simulink model "SPGF_FSK_0000_R2022b"  (R2022b)
settings: Solver=ode4  StartTime=0.0  StopTime=1.4  FixedStep=50e-6/50  RelTol=1e-3  EnableMultiTasking=on
undefined symbols (not defined in the file): D11, Delta
libraries: spsSeriesRLCBranchLib x1646, spsGroundLib x360, spsStairGeneratorLib x147, spsIdealSwitchLib x145, spsCurrentMeasurementLib x145, spsUniversalBridgeLib x76, spsThreePhaseSeriesRLCLoadLib x57, simulink x45, spsBistableLib x36, spsSequenceAnalyzerLib x31, spsThreePhaseParallelRLCLoadLib x20, spsThreePhaseTransformerTwoWindingsLib x20
(part 25 of 40)

== system SPGF_FSK_0000_R2022b/W33/DPL ==
  Ccs2/1 : spsSeriesRLCBranchLib/Series RLC Branch  LConnTagsString=__new0  RConnTagsString=__new0  BranchType=R  Resistance=-Rg_matrix(3,4)*2  Inductance=1e-3  SetiL0=off  InitialCurrent=0  Capacitance=Rg_matrix(3,4)*2  Setx0=off  InitialVoltage=0  Measurements=None
  Ccs2/3 : spsSeriesRLCBranchLib/Series RLC Branch  LConnTagsString=__new0  RConnTagsString=__new0  BranchType=R  Resistance=-Rg_matrix(3,4)*2  Inductance=1e-3  SetiL0=off  InitialCurrent=0  Capacitance=Rg_matrix(3,4)*2  Setx0=off  InitialVoltage=0  Measurements=None
  Ccs3/1 : spsSeriesRLCBranchLib/Series RLC Branch  LConnTagsString=__new0  RConnTagsString=__new0  BranchType=R  Resistance=-Rg_matrix(5,6)*2  Inductance=1e-3  SetiL0=off  InitialCurrent=0  Capacitance=-C_matrix(5,6)/2  Setx0=off  InitialVoltage=0  Measurements=None
  Ccs3/3 : spsSeriesRLCBranchLib/Series RLC Branch  LConnTagsString=__new0  RConnTagsString=__new0  BranchType=R  Resistance=-Rg_matrix(5,6)*2  Inductance=1e-3  SetiL0=off  InitialCurrent=0  Capacitance=-C_matrix(5,6)/2  Setx0=off  InitialVoltage=0  Measurements=None
  DPL : spsDistributedParametersLineLib/Distributed Parameters Line  Phases=6  Length=LineLength  Frequency=Frequency  Resistance=R_matrix  Inductance=L_matrix  Capacitance=C_matrix  x1=[-2.15e-05 -1.53051007031569 0 -12.0034457369496 0 0 -8990.94401290029;-2.1e-05 -1.53094778670127 0 -12.0068977094404 0 0 -8990.15397169475;-2.05e-05 -1.53138546531224 0 -12.010349385673 0 0 -8989.36370866606;-2e-05 -1.53182310613778 0 -12.013800765562 0 0 -8988.5732238337;-1.95e-05 -1.5322607091671 0 -12.0172518490225 0 0 -8987.78251721719;-1.9e-05 -1.5326982743894 0 -12.0207026359691 0 0 -8986.99158883604;-1.85e-05 -1.53313580179389 0 -12.0241531263167 0 0 -8986.20043870976;-1.8e-05 -1.53357329136977 0 -12.0276033199803 0 0 -8985.40906685787;-1.75e-05 -1.53401074310624 0 -12.0310532168746 0 0 -8984.6174732999;-1.7e-05 -1.53444815699252 0 -12.0345028169147 0 0 -8983.82565805538;-1.65e-05 -1.53488553301781 0 -12.0379521200152 0 0 -8983.03362114385;-1.6e-05 -1.53532287117131 0 -12.0414011260912 0 0 -8982.24136258485;-1.55e-05 -1.53576017144224 0 -12.0448498350576 0 0 -8981.44888239792;-1.5e-05 -1.53619743381981 0 -12.0482982468291 0 0 -8980.65618060263;-1.45e-05 -1.53663465829322 0 -12.0517463613209 0 0 -8979.86325721853;-1.4e-05 -1.5370718448517 0 -12.0551941784477 0 0 -8979.07011226518;-1.35e-05 -1.53750899348445 0 -12.0586416981245 0 0 -8978.27674576216;-1.3e-05 -1.53794610418068 0 -12.0620889202663 0 0 -8977.48315772904;-1.25e-05 -1.53838317692962 0 -12.0655358447879 0 0 -8976.68934818541;-1.2e-05 -1.53882021172047 0 -12.0689824716044 0 0 -8975.89531715084;-1.15e-05 -1.53925720854245 0 -12.0724288006307 0 0 -8975.10106464493;-1.1e-05 -1.53969416738479 0 -12.0758748317817 0 0 -8974.30659068728;-1.05e-05 -1.54013108823669 0 -12.0793205649725 0 0 -8973.51189529749;-1e-05 -1.54056797108738 0 -12.082766000118 0 0 -8972.71697849517;-9.5e-06 -1.54100481592609 0 -12.0862111371332 0 0 -8971.92184029994;-9e-06 -1.54144162274202 0 -12.089655975933 0 0 -8971.1264807314;-8.5e-06 -1.5418783915244 0 -12.0931005164326 0 0 -8970.33089980919;-8e-06 -1.54231512226246 0 -12.0965447585469 0 0 -8969.53509755294;-7.5e-06 -1.54275181494542 0 -12.0999887021909 0 0 -8968.73907398229;-7e-06 -1.54318846956251 0 -12.1034323472796 0 0 -8967.94282911686;-6.5e-06 -1.54362508610295 0 -12.1068756937282 0 0 -8967.14636297632;-6e-06 -1.54406166455596 0 -12.1103187414515 0 0 -8966.34967558031;-5.5e-06 -1.54449820491078 0 -12.1137614903647 0 0 -8965.55276694849;-5e-06 -1.54493470715663 0 -12.1172039403828 0 0 -8964.75563710052;-4.5e-06 -1.54537117128275 0 -12.1206460914209 0 0 -8963.95828605607;-4e-06 -1.54580759727836 0 -12.1240879433941 -2673.48580378537 0 -8963.16071383482;-3.5e-06 -1.5462439851327 5069.86085970959 -12.1275294962173 -2674.22835810835 4729.05893929821 -8962.36292045645;-3e-06 -1.546680334835 5071.26848541117 -12.1309707498058 -2674.97084644739 4728.63786087132 -8961.56490594063;-2.5e-06 -1.54711664637449 5072.67598598422 -12.1344117040746 -2675.71326878417 4728.21666576997 -8960.76667030706;-2e-06 -1.54755291974041 5074.08336139401 -12.1378523589387 -2676.45562510037 4727.79535400456 -8959.96821357544;-1.5e-06 -1.54798915492199 5075.49061160581 -12.1412927143134 -2677.19791537767 4727.37392558546 -8959.16953576546;-1e-06 -1.54842535190847 5076.8977365849 -12.1447327701137 -2677.94013959777 4726.9523805231 -8958.37063689683;-5e-07 -1.54886151068908 5078.30473629656 -12.1481725262546 -2678.68229774234 4726.53071882785 -8957.57151698927]  x2=[-2.15e-05 -1.52937369923623 0 -11.9860465797701 0 0 -9022.25103677801;-2.1e-05 -1.52981566216544 0 -11.9895391205462 0 0 -9021.46040632605;-2.05e-05 -1.53025758734796 0 -11.9930313654924 0 0 -9020.66955327848;-2e-05 -1.5306994747729 0 -11.9965233145224 0 0 -9019.87847765481;-1.95e-05 -1.53114132442933 0 -12.00001496755 0 0 -9019.08717947456;-1.9e-05 -1.53158313630637 0 -12.0035063244892 0 0 -9018.29565875726;-1.85e-05 -1.53202491039311 0 -12.0069973852536 0 0 -9017.50391552242;-1.8e-05 -1.53246664667865 0 -12.0104881497573 0 0 -9016.7119497896;-1.75e-05 -1.53290834515209 0 -12.0139786179141 0 0 -9015.91976157833;-1.7e-05 -1.53335000580254 0 -12.0174687896379 0 0 -9015.12735090815;-1.65e-05 -1.53379162861909 0 -12.0209586648425 0 0 -9014.33471779863;-1.6e-05 -1.53423321359085 0 -12.0244482434418 0 0 -9013.54186226931;-1.55e-05 -1.53467476070692 0 -12.0279375253497 0 0 -9012.74878433976;-1.5e-05 -1.5351162699564 0 -12.0314265104802 0 0 -9011.95548402955;-1.45e-05 -1.53555774132842 0 -12.0349151987472 0 0 -9011.16196135825;-1.4e-05 -1.53599917481206 0 -12.0384035900645 0 0 -9010.36821634544;-1.35e-05 -1.53644057039645 0 -12.0418916843461 0 0 -9009.57424901071;-1.3e-05 -1.53688192807068 0 -12.0453794815059 0 0 -9008.78005937364;-1.25e-05 -1.53732324782387 0 -12.0488669814579 0 0 -9007.98564745383;-1.2e-05 -1.53776452964513 0 -12.0523541841161 0 0 -9007.19101327089;-1.15e-05 -1.53820577352357 0 -12.0558410893943 0 0 -9006.39615684442;-1.1e-05 -1.53864697944831 0 -12.0593276972066 0 0 -9005.60107819403;-1.05e-05 -1.53908814740845 0 -12.0628140074669 0 0 -9004.80577733934;-1e-05 -1.53952927739312 0 -12.0663000200891 0 0 -9004.01025429998;-9.5e-06 -1.53997036939142 0 -12.0697857349874 0 0 -9003.21450909557;-9e-06 -1.54041142339248 0 -12.0732711520756 0 0 -9002.41854174574;-8.5e-06 -1.54085243938541 0 -12.0767562712678 0 0 -9001.62235227014;-8e-06 -1.54129341735933 0 -12.080241092478 0 0 -9000.82594068841;-7.5e-06 -1.54173435730336 0 -12.0837256156202 0 0 -9000.02930702021;-7e-06 -1.54217525920661 0 -12.0872098406084 0 0 -8999.23245128518;-6.5e-06 -1.54261612305822 0 -12.0906937673567 0 0 -8998.43537350299;-6e-06 -1.5430569488473 0 -12.0941773957791 0 0 -8997.63807369331;-5.5e-06 -1.54349773656298 0 -12.0976607257895 0 0 -8996.84055187581;-5e-06 -1.54393848619438 0 -12.1011437573022 0 0 -8996.04280807017;-4.5e-06 -1.54437919773062 0 -12.1046264902311 0 0 -8995.24484229607;-4e-06 -1.54481987116083 0 -12.1081089244904 -2677.09103389761 0 -8994.4466545732;-3.5e-06 -1.54526050647415 5076.70076594894 -12.111591059994 -2677.83624236647 4745.56687862651 -8993.64824492125;-3e-06 -1.54570110365968 5078.11342326981 -12.1150728966561 -2678.58138476238 4745.14547461087 -8992.84961335993;-2.5e-06 -1.54614166270657 5079.52595529325 -12.1185544343908 -2679.32646106693 4744.72395351346 -8992.05075990894;-2e-06 -1.54658218360395 5080.93836198442 -12.1220356731121 -2680.07147126176 4744.30231534468 -8991.25168458799;-1.5e-06 -1.54702266634093 5082.35064330845 -12.1255166127341 -2680.81641532848 4743.88056011494 -8990.45238741679;-1e-06 -1.54746311090667 5083.76279923051 -12.1289972531711 -2681.5612932487 4743.45868783463 -8989.65286841508;-5e-07 -1.54790351729028 5085.17482971575 -12.132477594337 -2682.30610500404 4743.03669851417 -8988.85312760257]  x3=[-2.15e-05 0.0136787460671286 0 -0.564718131480657 0 0 -283.556160613102;-2.1e-05 0.0136746389724756 0 -0.565073370432723 0 0 -283.549477726857;-2.05e-05 0.0136705315404145 0 -0.565428595442164 0 0 -283.542787844309;-2e-05 0.0136664237710464 0 -0.565783806500213 0 0 -283.536090965623;-1.95e-05 0.0136623156644729 0 -0.566139003598106 0 0 -283.529387090964;-1.9e-05 0.0136582072207953 0 -0.566494186727079 0 0 -283.522676220498;-1.85e-05 0.0136540984401149 0 -0.566849355878369 0 0 -283.515958354391;-1.8e-05 0.0136499893225332 0 -0.567204511043211 0 0 -283.509233492808;-1.75e-05 0.0136458798681514 0 -0.567559652212843 0 0 -283.502501635915;-1.7e-05 0.0136417700770711 0 -0.567914779378502 0 0 -283.495762783878;-1.65e-05 0.0136376599493936 0 -0.568269892531425 0 0 -283.489016936863;-1.6e-05 0.0136335494852203 0 -0.568624991662851 0 0 -283.482264095037;-1.55e-05 0.0136294386846526 0 -0.568980076764017 0 0 -283.475504258567;-1.5e-05 0.0136253275477921 0 -0.569335147826163 0 0 -283.468737427619;-1.45e-05 0.01362121607474 0 -0.569690204840527 0 0 -283.461963602361;-1.4e-05 0.013617104265598 0 -0.570045247798349 0 0 -283.455182782959;-1.35e-05 0.0136129921204673 0 -0.570400276690868 0 0 -283.44839496958;-1.3e-05 0.0136088796394495 0 -0.570755291509325 0 0 -283.441600162393;-1.25e-05 0.0136047668226461 0 -0.571110292244959 0 0 -283.434798361565;-1.2e-05 0.0136006536701585 0 -0.571465278889011 0 0 -283.427989567263;-1.15e-05 0.0135965401820883 0 -0.571820251432724 0 0 -283.421173779656;-1.1e-05 0.0135924263585368 0 -0.572175209867336 0 0 -283.414350998912;-1.05e-05 0.0135883121996057 0 -0.572530154184092 0 0 -283.407521225199;-1e-05 0.0135841977053964 0 -0.572885084374232 0 0 -283.400684458686;-9.5e-06 0.0135800828760105 0 -0.573240000428999 0 0 -283.393840699541;-9e-06 0.0135759677115495 0 -0.573594902339637 0 0 -283.386989947933;-8.5e-06 0.0135718522121149 0 -0.573949790097387 0 0 -283.380132204032;-8e-06 0.0135677363778082 0 -0.574304663693494 0 0 -283.373267468006;-7.5e-06 0.0135636202087311 0 -0.574659523119202 0 0 -283.366395740025;-7e-06 0.0135595037049851 0 -0.575014368365753 0 0 -283.359517020259;-6.5e-06 0.0135553868666717 0 -0.575369199424395 0 0 -283.352631308877;-6e-06 0.0135512696938925 0 -0.57572401628637 0 0 -283.345738606048;-5.5e-06 0.0135471521867492 0 -0.576078818942925 0 0 -283.338838911944;-5e-06 0.0135430343453433 0 -0.576433607385304 0 0 -283.331932226735;-4.5e-06 0.0135389161697764 0 -0.576788381604755 0 0 -283.32501855059;-4e-06 0.0135347976601502 0 -0.577143141592522 -226.331790311316 0 -283.31809788368;-3.5e-06 0.0135306788165662 30.8698318235783 -0.577497887339853 -226.40077511491 467.902729417475 -283.311170226177;-3e-06 0.0135265596391261 30.9112443496022 -0.577852618837996 -226.469754332289 467.86511811605 -283.304235578251;-2.5e-06 0.0135224401279315 30.9526561129216 -0.578207336078196 -226.538727961751 467.827495270517 -283.297293940073;-2e-06 0.0135183202830841 30.994067112515 -0.578562039051702 -226.607696001593 467.789860881802 -283.290345311814;-1.5e-06 0.0135142001046855 31.0354773473603 -0.578916727749762 -226.676658450115 467.752214950836 -283.283389693647;-1e-06 0.0135100795928374 31.076886816436 -0.579271402163624 -226.745615305614 467.714557478546 -283.276427085742;-5e-07 0.0135059587476414 31.1182955187202 -0.579626062284538 -226.81456656639 467.676888465862 -283.269457488271]  x4=[-2.15e-05 -0.0335597763976248 0 -0.864079445727117 0 0 19.5995628520039;-2.1e-05 -0.0335614302550886 0 -0.864138531180508 0 0 19.6160167362686;-2.05e-05 -0.0335630832844574 0 -0.864197595312135 0 0 19.6324701365274;-2e-05 -0.0335647354856902 0 -0.864256638120542 0 0 19.6489230523744;-1.95e-05 -0.0335663868587464 0 -0.864315659604271 0 0 19.6653754834037;-1.9e-05 -0.0335680374035852 0 -0.864374659761866 0 0 19.6818274292093;-1.85e-05 -0.0335696871201659 0 -0.864433638591871 0 0 19.6982788893853;-1.8e-05 -0.0335713360084478 0 -0.864492596092831 0 0 19.7147298635258;-1.75e-05 -0.0335729840683902 0 -0.864551532263291 0 0 19.7311803512247;-1.7e-05 -0.0335746312999523 0 -0.864610447101797 0 0 19.7476303520763;-1.65e-05 -0.0335762777030937 0 -0.864669340606895 0 0 19.7640798656747;-1.6e-05 -0.0335779232777736 0 -0.864728212777133 0 0 19.7805288916139;-1.55e-05 -0.0335795680239515 0 -0.864787063611058 0 0 19.7969774294882;-1.5e-05 -0.0335812119415867 0 -0.864845893107216 0 0 19.8134254788916;-1.45e-05 -0.0335828550306387 0 -0.864904701264158 0 0 19.8298730394183;-1.4e-05 -0.0335844972910671 0 -0.864963488080432 0 0 19.8463201106626;-1.35e-05 -0.0335861387228311 0 -0.865022253554587 0 0 19.8627666922185;-1.3e-05 -0.0335877793258904 0 -0.865080997685174 0 0 19.8792127836803;-1.25e-05 -0.0335894191002045 0 -0.865139720470742 0 0 19.8956583846421;-1.2e-05 -0.0335910580457328 0 -0.865198421909844 0 0 19.9121034946983;-1.15e-05 -0.0335926961624351 0 -0.86525710200103 0 0 19.9285481134431;-1.1e-05 -0.0335943334502708 0 -0.865315760742853 0 0 19.9449922404706;-1.05e-05 -0.0335959699091995 0 -0.865374398133866 0 0 19.9614358753751;-1e-05 -0.0335976055391809 0 -0.865433014172621 0 0 19.977879017751;-9.5e-06 -0.0335992403401746 0 -0.865491608857673 0 0 19.9943216671924;-9e-06 -0.0336008743121403 0 -0.865550182187575 0 0 20.0107638232938;-8.5e-06 -0.0336025074550377 0 -0.865608734160882 0 0 20.0272054856493;-8e-06 -0.0336041397688264 0 -0.86566726477615 0 0 20.0436466538534;-7.5e-06 -0.0336057712534662 0 -0.865725774031935 0 0 20.0600873275003;-7e-06 -0.0336074019089168 0 -0.865784261926792 0 0 20.0765275061844;-6.5e-06 -0.0336090317351381 0 -0.865842728459279 0 0 20.0929671895;-6e-06 -0.0336106607320897 0 -0.865901173627952 0 0 20.1094063770415;-5.5e-06 -0.0336122888997315 0 -0.865959597431371 0 0 20.1258450684033;-5e-06 -0.0336139162380233 0 -0.866017999868093 0 0 20.1422832631798;-4.5e-06 -0.033615542746925 0 -0.866076380936678 0 0 20.1587209609654;-4e-06 -0.0336171684263964 0 -0.866134740635685 -208.15535285938 0 20.1751581613545;-3.5e-06 -0.0336187932763974 96.5153015550597 -0.866193078963673 -208.207336373204 362.803625462547 20.1915948639415;-3e-06 -0.033620417296888 96.5093417255004 -0.866251395919204 -208.259314749717 362.767458802469 20.2080310683209;-2.5e-06 -0.033622040487828 96.5033795146685 -0.866309691500839 -208.311287987638 362.731283191463 20.2244667740871;-2e-06 -0.0336236628491774 96.4974149227112 -0.866367965707138 -208.363256085684 362.695098630421 20.2409019808345;-1.5e-06 -0.0336252843808962 96.4914479497756 -0.866426218536665 -208.415219042573 362.658905120237 20.2573366881578;-1e-06 -0.0336269050829444 96.485478596009 -0.866484449987982 -208.467176857022 362.622702661802 20.2737708956513;-5e-07 -0.0336285249552819 96.4795068615586 -0.866542660059652 -208.51912952775 362.586491256011 20.2902046029095]  x5=2.11324941411031e-05  V1=ones(3,3)  V2=ones(3,3)  I1=ones(3,3)  I2=ones(3,3)  nHarmo=1  Measurements=None  Decoupling=off  VsMag0=0  VrMag0=0  VsAngle0=0  VrAngle0=0  IsMag0=0  IrMag0=0  IsAngle0=0  IrAngle0=0
      settings: LibrarySourceBlock=sps_lib/Power Grid Elements/Distributed Parameters Line
  Ground{1..4} (4 alike) : spsGroundLib/Ground  LConnTagsString=a
  Rcs*1 : spsSeriesRLCBranchLib/Series RLC Branch  LConnTagsString=__new0  RConnTagsString=__new0  BranchType=R  Resistance=-Rg_matrix(1,2)*2  Inductance=1e-3  SetiL0=off  InitialCurrent=0  Capacitance=Rg_matrix(1,2)*2  Setx0=off  InitialVoltage=0  Measurements=None
  Rcs*2 : spsSeriesRLCBranchLib/Series RLC Branch  LConnTagsString=__new0  RConnTagsString=__new0  BranchType=R  Resistance=-Rg_matrix(1,2)*2  Inductance=1e-3  SetiL0=off  InitialCurrent=0  Capacitance=Rg_matrix(1,2)*2  Setx0=off  InitialVoltage=0  Measurements=None
  Rgsg1/1 : spsSeriesRLCBranchLib/Series RLC Branch  LConnTagsString=__new0  RConnTagsString=__new0  BranchType=R  Resistance=(Rg_matrix(4,4)+Rg_matrix(3,4))*2  Inductance=1e-3  SetiL0=off  InitialCurrent=0  Capacitance=Rg_matrix(1,2)*2  Setx0=off  InitialVoltage=0  Measurements=None
  Rgsg1/2 : spsSeriesRLCBranchLib/Series RLC Branch  LConnTagsString=__new0  RConnTagsString=__new0  BranchType=R  Resistance=(Rg_matrix(2,2)+Rg_matrix(1,2))*2  Inductance=1e-3  SetiL0=off  InitialCurrent=0  Capacitance=Rg_matrix(1,2)*2  Setx0=off  InitialVoltage=0  Measurements=None
  Rgsg1/3 : spsSeriesRLCBranchLib/Series RLC Branch  LConnTagsString=__new0  RConnTagsString=__new0  BranchType=R  Resistance=(Rg_matrix(4,4)+Rg_matrix(3,4))*2  Inductance=1e-3  SetiL0=off  InitialCurrent=0  Capacitance=Rg_matrix(1,2)*2  Setx0=off  InitialVoltage=0  Measurements=None
  Rgsg1/4 : spsSeriesRLCBranchLib/Series RLC Branch  LConnTagsString=__new0  RConnTagsString=__new0  BranchType=R  Resistance=(Rg_matrix(2,2)+Rg_matrix(1,2))*2  Inductance=1e-3  SetiL0=off  InitialCurrent=0  Capacitance=Rg_matrix(1,2)*2  Setx0=off  InitialVoltage=0  Measurements=None
  Rsg*1 : spsSeriesRLCBranchLib/Series RLC Branch  LConnTagsString=__new0  RConnTagsString=__new0  BranchType=R  Resistance=(Rg_matrix(6,6)+Rg_matrix(5,6))*2  Inductance=1e-3  SetiL0=off  InitialCurrent=0  Capacitance=Rg_matrix(1,2)*2  Setx0=off  InitialVoltage=0  Measurements=None
  Rsg*2 : spsSeriesRLCBranchLib/Series RLC Branch  LConnTagsString=__new0  RConnTagsString=__new0  BranchType=R  Resistance=(Rg_matrix(6,6)+Rg_matrix(5,6))*2  Inductance=1e-3  SetiL0=off  InitialCurrent=0  Capacitance=Rg_matrix(1,2)*2  Setx0=off  InitialVoltage=0  Measurements=None
  A : PMIOPort  Side=Left
  B : PMIOPort  Port=2  Side=Left
  C : PMIOPort  Port=3  Side=Left
  a : PMIOPort  Port=4  Side=Right
  b : PMIOPort  Port=5  Side=Right
  c : PMIOPort  Port=6  Side=Right
  connections:
  A/RConn1 -- DPL/LConn1 -- Rcs*2/RConn1
  B/RConn1 -- DPL/LConn3 -- Ccs2/3/RConn1
  C/RConn1 -- DPL/LConn5 -- Ccs3/3/RConn1
  Rgsg1/2/RConn1 -- Rsg*2/RConn1 -- Rgsg1/1/RConn1 -- Ground2/LConn1
  DPL/LConn2 -- Rcs*2/LConn1 -- Rgsg1/2/LConn1 -- DPL/LConn4 -- Ccs2/3/LConn1 -- Rgsg1/1/LConn1 -- DPL/LConn6 -- Rsg*2/LConn1 -- Ccs3/3/LConn1 -- Ground3/LConn1
  Rgsg1/3/RConn1 -- Rsg*1/RConn1 -- Rgsg1/4/RConn1 -- Ground1/LConn1
  Rgsg1/3/LConn1 -- Ccs2/1/LConn1 -- DPL/RConn4 -- DPL/RConn2 -- Rgsg1/4/LConn1 -- Rcs*1/LConn1 -- Rsg*1/LConn1 -- Ccs3/1/LConn1 -- DPL/RConn6 -- Ground4/LConn1
  Rcs*1/RConn1 -- DPL/RConn1 -- a/RConn1
  DPL/RConn3 -- Ccs2/1/RConn1 -- b/RConn1
  DPL/RConn5 -- Ccs3/1/RConn1 -- c/RConn1

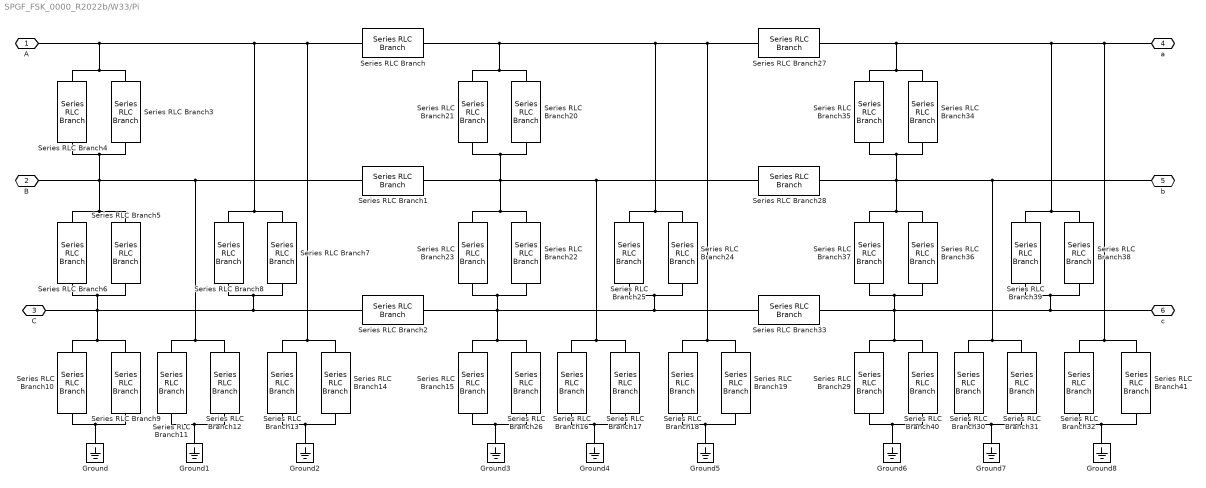
== system SPGF_FSK_0000_R2022b/W33/Pi ==
  Ground{,1..8} (9 alike) : spsGroundLib/Ground  LConnTagsString=a
  Series RLC Branch{,1..2,27..28,33} (6 alike) : spsSeriesRLCBranchLib/Series RLC Branch  LConnTagsString=__new0  RConnTagsString=__new0  BranchType=RL  Resistance=R/2  Inductance=L/2  SetiL0=off  InitialCurrent=0  Capacitance=1e-6  Setx0=off  InitialVoltage=0  Measurements=None
  Series RLC Branch{10..11,13,29..30,32} (6 alike) : spsSeriesRLCBranchLib/Series RLC Branch  LConnTagsString=__new0  RConnTagsString=__new0  BranchType=R  Resistance=Rfg*4  Inductance=L/2  SetiL0=off  InitialCurrent=0  Capacitance=1e-6  Setx0=off  InitialVoltage=0  Measurements=None
  Series RLC Branch{9,12,14,31,40..41} (6 alike) : spsSeriesRLCBranchLib/Series RLC Branch  LConnTagsString=__new0  RConnTagsString=__new0  BranchType=C  Resistance=R/2  Inductance=L/2  SetiL0=off  InitialCurrent=0  Capacitance=Cfg*0.25  Setx0=off  InitialVoltage=0  Measurements=None
  Series RLC Branch15 : spsSeriesRLCBranchLib/Series RLC Branch  LConnTagsString=__new0  RConnTagsString=__new0  BranchType=R  Resistance=Rfg*2  Inductance=L/2  SetiL0=off  InitialCurrent=0  Capacitance=1e-6  Setx0=off  InitialVoltage=0  Measurements=None
  Series RLC Branch16 : spsSeriesRLCBranchLib/Series RLC Branch  LConnTagsString=__new0  RConnTagsString=__new0  BranchType=R  Resistance=Rfg*2  Inductance=L/2  SetiL0=off  InitialCurrent=0  Capacitance=1e-6  Setx0=off  InitialVoltage=0  Measurements=None
  Series RLC Branch17 : spsSeriesRLCBranchLib/Series RLC Branch  LConnTagsString=__new0  RConnTagsString=__new0  BranchType=C  Resistance=R/2  Inductance=L/2  SetiL0=off  InitialCurrent=0  Capacitance=Cfg*0.5  Setx0=off  InitialVoltage=0  Measurements=None
  Series RLC Branch18 : spsSeriesRLCBranchLib/Series RLC Branch  LConnTagsString=__new0  RConnTagsString=__new0  BranchType=R  Resistance=Rfg*2  Inductance=L/2  SetiL0=off  InitialCurrent=0  Capacitance=1e-6  Setx0=off  InitialVoltage=0  Measurements=None
  Series RLC Branch19 : spsSeriesRLCBranchLib/Series RLC Branch  LConnTagsString=__new0  RConnTagsString=__new0  BranchType=C  Resistance=R/2  Inductance=L/2  SetiL0=off  InitialCurrent=0  Capacitance=Cfg*0.5  Setx0=off  InitialVoltage=0  Measurements=None
  Series RLC Branch20 : spsSeriesRLCBranchLib/Series RLC Branch  LConnTagsString=__new0  RConnTagsString=__new0  BranchType=C  Resistance=R/2  Inductance=L/2  SetiL0=off  InitialCurrent=0  Capacitance=Cmf*0.5  Setx0=off  InitialVoltage=0  Measurements=None
  Series RLC Branch21 : spsSeriesRLCBranchLib/Series RLC Branch  LConnTagsString=__new0  RConnTagsString=__new0  BranchType=R  Resistance=Rmf*2  Inductance=L/2  SetiL0=off  InitialCurrent=0  Capacitance=1e-6  Setx0=off  InitialVoltage=0  Measurements=None
  Series RLC Branch22 : spsSeriesRLCBranchLib/Series RLC Branch  LConnTagsString=__new0  RConnTagsString=__new0  BranchType=C  Resistance=R/2  Inductance=L/2  SetiL0=off  InitialCurrent=0  Capacitance=Cmf*0.5  Setx0=off  InitialVoltage=0  Measurements=None
  Series RLC Branch23 : spsSeriesRLCBranchLib/Series RLC Branch  LConnTagsString=__new0  RConnTagsString=__new0  BranchType=R  Resistance=Rmf*2  Inductance=L/2  SetiL0=off  InitialCurrent=0  Capacitance=1e-6  Setx0=off  InitialVoltage=0  Measurements=None
  Series RLC Branch24 : spsSeriesRLCBranchLib/Series RLC Branch  LConnTagsString=__new0  RConnTagsString=__new0  BranchType=C  Resistance=R/2  Inductance=L/2  SetiL0=off  InitialCurrent=0  Capacitance=Cmf*0.5  Setx0=off  InitialVoltage=0  Measurements=None
  Series RLC Branch25 : spsSeriesRLCBranchLib/Series RLC Branch  LConnTagsString=__new0  RConnTagsString=__new0  BranchType=R  Resistance=Rmf*2  Inductance=L/2  SetiL0=off  InitialCurrent=0  Capacitance=1e-6  Setx0=off  InitialVoltage=0  Measurements=None
  Series RLC Branch26 : spsSeriesRLCBranchLib/Series RLC Branch  LConnTagsString=__new0  RConnTagsString=__new0  BranchType=C  Resistance=R/2  Inductance=L/2  SetiL0=off  InitialCurrent=0  Capacitance=Cfg*0.5  Setx0=off  InitialVoltage=0  Measurements=None
  Series RLC Branch{3,5,7,34,36,38} (6 alike) : spsSeriesRLCBranchLib/Series RLC Branch  LConnTagsString=__new0  RConnTagsString=__new0  BranchType=C  Resistance=R/2  Inductance=L/2  SetiL0=off  InitialCurrent=0  Capacitance=Cmf*0.25  Setx0=off  InitialVoltage=0  Measurements=None
  Series RLC Branch{4,6,8,35,37,39} (6 alike) : spsSeriesRLCBranchLib/Series RLC Branch  LConnTagsString=__new0  RConnTagsString=__new0  BranchType=R  Resistance=Rmf*4  Inductance=L/2  SetiL0=off  InitialCurrent=0  Capacitance=1e-6  Setx0=off  InitialVoltage=0  Measurements=None
  A : PMIOPort  Side=Left
  B : PMIOPort  Port=2  Side=Left
  C : PMIOPort  Port=3  Side=Left
  a : PMIOPort  Port=4  Side=Right
  b : PMIOPort  Port=5  Side=Right
  c : PMIOPort  Port=6  Side=Right
  connections:
  Series RLC Branch12/LConn1 -- Series RLC Branch11/LConn1 -- Series RLC Branch5/LConn1 -- Series RLC Branch6/LConn1 -- B/RConn1 -- Series RLC Branch4/RConn1 -- Series RLC Branch3/RConn1 -- Series RLC Branch1/LConn1
  Series RLC Branch13/LConn1 -- A/RConn1 -- Series RLC Branch4/LConn1 -- Series RLC Branch3/LConn1 -- Series RLC Branch7/LConn1 -- Series RLC Branch8/LConn1 -- Series RLC Branch/LConn1 -- Series RLC Branch14/LConn1
  Series RLC Branch9/LConn1 -- Series RLC Branch2/LConn1 -- Series RLC Branch8/RConn1 -- Series RLC Branch7/RConn1 -- C/RConn1 -- Series RLC Branch5/RConn1 -- Series RLC Branch6/RConn1 -- Series RLC Branch10/LConn1
  Series RLC Branch9/RConn1 -- Ground/LConn1 -- Series RLC Branch10/RConn1
  Series RLC Branch12/RConn1 -- Series RLC Branch11/RConn1 -- Ground1/LConn1
  Series RLC Branch13/RConn1 -- Series RLC Branch14/RConn1 -- Ground2/LConn1
  Series RLC Branch17/LConn1 -- Series RLC Branch16/LConn1 -- Series RLC Branch28/LConn1 -- Series RLC Branch1/RConn1 -- Series RLC Branch23/LConn1 -- Series RLC Branch22/LConn1 -- Series RLC Branch20/RConn1 -- Series RLC Branch21/RConn1
  Series RLC Branch21/LConn1 -- Series RLC Branch20/LConn1 -- Series RLC Branch/RConn1 -- Series RLC Branch27/LConn1 -- Series RLC Branch19/LConn1 -- Series RLC Branch18/LConn1 -- Series RLC Branch24/LConn1 -- Series RLC Branch25/LConn1
  Series RLC Branch26/LConn1 -- Series RLC Branch15/LConn1 -- Series RLC Branch2/RConn1 -- Series RLC Branch33/LConn1 -- Series RLC Branch25/RConn1 -- Series RLC Branch24/RConn1 -- Series RLC Branch22/RConn1 -- Series RLC Branch23/RConn1
  Series RLC Branch26/RConn1 -- Series RLC Branch15/RConn1 -- Ground3/LConn1
  Ground4/LConn1 -- Series RLC Branch17/RConn1 -- Series RLC Branch16/RConn1
  Ground5/LConn1 -- Series RLC Branch18/RConn1 -- Series RLC Branch19/RConn1
  Series RLC Branch31/LConn1 -- b/RConn1 -- Series RLC Branch35/RConn1 -- Series RLC Branch34/RConn1 -- Series RLC Branch36/LConn1 -- Series RLC Branch37/LConn1 -- Series RLC Branch28/RConn1 -- Series RLC Branch30/LConn1
  Series RLC Branch34/LConn1 -- a/RConn1 -- Series RLC Branch41/LConn1 -- Series RLC Branch32/LConn1 -- Series RLC Branch38/LConn1 -- Series RLC Branch39/LConn1 -- Series RLC Branch27/RConn1 -- Series RLC Branch35/LConn1
  Series RLC Branch29/LConn1 -- Series RLC Branch36/RConn1 -- Series RLC Branch37/RConn1 -- c/RConn1 -- Series RLC Branch39/RConn1 -- Series RLC Branch38/RConn1 -- Series RLC Branch33/RConn1 -- Series RLC Branch40/LConn1
  Series RLC Branch29/RConn1 -- Series RLC Branch40/RConn1 -- Ground6/LConn1
  Series RLC Branch31/RConn1 -- Series RLC Branch30/RConn1 -- Ground7/LConn1
  Series RLC Branch32/RConn1 -- Series RLC Branch41/RConn1 -- Ground8/LConn1

== system SPGF_FSK_0000_R2022b/W33/Q ==
  breaker : Subsystem  Commented=on  mask{SwitchA=off, SwitchB=off, SwitchC=off, InitialStatus=[1 1 1], BreakerResistance=0.0001, SnubberResistance=1e6, SnubberCapacitance=inf, TransitionTimes=[0.5 0.7], ShiftTimes=[0 0 0]}
      mask prompts: SwitchA "Switching of phase A"; SwitchB "Switching of phase B"; SwitchC "Switching of phase C"; InitialStatus "Initial status of phase breaker [A, B, C]"; BreakerResistance "Breaker resistance Ron (ohms) :"; SnubberResistance "Snubbers resistance Rp (ohms) :"; SnubberCapacitance "Snubbers capacitance Cp (F) :"; TransitionTimes "Transition times (s) :"; ShiftTimes "Time differences for switch [tA, tB, tC] (s) :"
      mask init: same as SPGF_FSK_0000_R2022b/Feed/Q/breaker
      mask Display:
      | % port_label('input',1,'Iabc');
      | 
      | port_label('lconn',1,'A');
      | port_label('lconn',2,'B');
      | port_label('lconn',3,'C');
      | 
      | port_label('rconn',1,'a');
      | port_label('rconn',2,'b');
      | port_label('rconn',3,'c');
      | 
      | disp('   Q    ');
  meas : Subsystem
  shunt : Subsystem
  A : PMIOPort  Side=Right
  B : PMIOPort  Port=2  Side=Right
  C : PMIOPort  Port=3  Side=Right
  a : PMIOPort  Port=4  Side=Left
  b : PMIOPort  Port=5  Side=Left
  c : PMIOPort  Port=6  Side=Left
  connections:
  shunt/LConn3 -- C/RConn1 -- breaker/LConn3
  shunt/LConn2 -- B/RConn1 -- breaker/LConn2
  A/RConn1 -- shunt/LConn1 -- breaker/LConn1
  meas/RConn1 -- a/RConn1
  meas/RConn2 -- b/RConn1
  meas/RConn3 -- c/RConn1
  meas/LConn3 -- breaker/RConn3 -- shunt/RConn3
  meas/LConn2 -- breaker/RConn2 -- shunt/RConn2
  meas/LConn1 -- breaker/RConn1 -- shunt/RConn1

== system SPGF_FSK_0000_R2022b/W33/concentrated ==
  Ccs/1 : spsSeriesRLCBranchLib/Series RLC Branch  LConnTagsString=__new0  RConnTagsString=__new0  BranchType=C  Resistance=190  Inductance=1e-3  SetiL0=off  InitialCurrent=0  Capacitance=-C_matrix(1,2)/2  Setx0=off  InitialVoltage=0  Measurements=None
  Ccs/2 : spsSeriesRLCBranchLib/Series RLC Branch  LConnTagsString=__new0  RConnTagsString=__new0  BranchType=C  Resistance=190  Inductance=1e-3  SetiL0=off  InitialCurrent=0  Capacitance=-C_matrix(1,2)/2  Setx0=off  InitialVoltage=0  Measurements=None
  Ccs2/1 : spsSeriesRLCBranchLib/Series RLC Branch  LConnTagsString=__new0  RConnTagsString=__new0  BranchType=C  Resistance=190  Inductance=1e-3  SetiL0=off  InitialCurrent=0  Capacitance=-C_matrix(3,4)/2  Setx0=off  InitialVoltage=0  Measurements=None
  Ccs2/2 : spsSeriesRLCBranchLib/Series RLC Branch  LConnTagsString=__new0  RConnTagsString=__new0  BranchType=C  Resistance=190  Inductance=1e-3  SetiL0=off  InitialCurrent=0  Capacitance=-C_matrix(3,4)/2  Setx0=off  InitialVoltage=0  Measurements=None
  Ccs2/3 : spsSeriesRLCBranchLib/Series RLC Branch  LConnTagsString=__new0  RConnTagsString=__new0  BranchType=R  Resistance=-Rg_matrix(3,4)*2  Inductance=1e-3  SetiL0=off  InitialCurrent=0  Capacitance=Rg_matrix(3,4)*2  Setx0=off  InitialVoltage=0  Measurements=None
  Ccs2/4 : spsSeriesRLCBranchLib/Series RLC Branch  LConnTagsString=__new0  RConnTagsString=__new0  BranchType=R  Resistance=-Rg_matrix(3,4)*2  Inductance=1e-3  SetiL0=off  InitialCurrent=0  Capacitance=Rg_matrix(3,4)*2  Setx0=off  InitialVoltage=0  Measurements=None
  Ccs3/1 : spsSeriesRLCBranchLib/Series RLC Branch  LConnTagsString=__new0  RConnTagsString=__new0  BranchType=C  Resistance=190  Inductance=1e-3  SetiL0=off  InitialCurrent=0  Capacitance=-C_matrix(5,6)/2  Setx0=off  InitialVoltage=0  Measurements=None
  Ccs3/2 : spsSeriesRLCBranchLib/Series RLC Branch  LConnTagsString=__new0  RConnTagsString=__new0  BranchType=C  Resistance=190  Inductance=1e-3  SetiL0=off  InitialCurrent=0  Capacitance=-C_matrix(5,6)/2  Setx0=off  InitialVoltage=0  Measurements=None
  Ccs3/3 : spsSeriesRLCBranchLib/Series RLC Branch  LConnTagsString=__new0  RConnTagsString=__new0  BranchType=R  Resistance=-Rg_matrix(5,6)*2  Inductance=1e-3  SetiL0=off  InitialCurrent=0  Capacitance=-C_matrix(5,6)/2  Setx0=off  InitialVoltage=0  Measurements=None
  Ccs3/4 : spsSeriesRLCBranchLib/Series RLC Branch  LConnTagsString=__new0  RConnTagsString=__new0  BranchType=R  Resistance=-Rg_matrix(5,6)*2  Inductance=1e-3  SetiL0=off  InitialCurrent=0  Capacitance=-C_matrix(5,6)/2  Setx0=off  InitialVoltage=0  Measurements=None
  Csg/2 : spsSeriesRLCBranchLib/Series RLC Branch  LConnTagsString=__new0  RConnTagsString=__new0  BranchType=C  Resistance=190  Inductance=1e-3  SetiL0=off  InitialCurrent=0  Capacitance=( C_matrix(1,2) + C_matrix(2,2) )/2  Setx0=off  InitialVoltage=0  Measurements=None
  Csg1/1 : spsSeriesRLCBranchLib/Series RLC Branch  LConnTagsString=__new0  RConnTagsString=__new0  BranchType=C  Resistance=190  Inductance=1e-3  SetiL0=off  InitialCurrent=0  Capacitance=( C_matrix(1,2) + C_matrix(2,2) )/2  Setx0=off  InitialVoltage=0  Measurements=None
  Csg2/1 : spsSeriesRLCBranchLib/Series RLC Branch  LConnTagsString=__new0  RConnTagsString=__new0  BranchType=C  Resistance=190  Inductance=1e-3  SetiL0=off  InitialCurrent=0  Capacitance=( C_matrix(3,4) + C_matrix(4,4) )/2  Setx0=off  InitialVoltage=0  Measurements=None
  Csg2/2 : spsSeriesRLCBranchLib/Series RLC Branch  LConnTagsString=__new0  RConnTagsString=__new0  BranchType=C  Resistance=190  Inductance=1e-3  SetiL0=off  InitialCurrent=0  Capacitance=( C_matrix(3,4) + C_matrix(4,4) )/2  Setx0=off  InitialVoltage=0  Measurements=None
  Csg3/1 : spsSeriesRLCBranchLib/Series RLC Branch  LConnTagsString=__new0  RConnTagsString=__new0  BranchType=C  Resistance=190  Inductance=1e-3  SetiL0=off  InitialCurrent=0  Capacitance=( C_matrix(5,6) + C_matrix(6,6) ) /2  Setx0=off  InitialVoltage=0  Measurements=None
  Csg3/2 : spsSeriesRLCBranchLib/Series RLC Branch  LConnTagsString=__new0  RConnTagsString=__new0  BranchType=C  Resistance=190  Inductance=1e-3  SetiL0=off  InitialCurrent=0  Capacitance=( C_matrix(5,6) + C_matrix(6,6) ) /2  Setx0=off  InitialVoltage=0  Measurements=None
  Ground{1..4} (4 alike) : spsGroundLib/Ground  LConnTagsString=a
  RL : spsMutualInductanceLib/Mutual Inductance  LConnTagsString=a|b|c|L4|L5|L6  RConnTagsString=A|B|C|R4|R5|R6  TypeOfMutual=Generalized mutual inductance  NumberOfWindings=6  SelfImpedance1=[1.1 1.1e-03]  SelfImpedance2=[ 1.1 1.1e-03]  ThreeWindings=on  SelfImpedance3=[ 1.1 1.1e-03]  MutualImpedance=[1.0 1.0e-03]  InductanceMatrix=L_matrix  ResistanceMatrix=R_matrix  Measurements=None
      settings: LibrarySourceBlock=sps_lib/Passives/Mutual Inductance
  Rcs*2 : spsSeriesRLCBranchLib/Series RLC Branch  LConnTagsString=__new0  RConnTagsString=__new0  BranchType=R  Resistance=-Rg_matrix(1,2)*2  Inductance=1e-3  SetiL0=off  InitialCurrent=0  Capacitance=Rg_matrix(1,2)*2  Setx0=off  InitialVoltage=0  Measurements=None
  Rgcs1/1 : spsSeriesRLCBranchLib/Series RLC Branch  LConnTagsString=__new0  RConnTagsString=__new0  BranchType=R  Resistance=-Rg_matrix(1,2)*2  Inductance=1e-3  SetiL0=off  InitialCurrent=0  Capacitance=Rg_matrix(1,2)*2  Setx0=off  InitialVoltage=0  Measurements=None
  Rgsg1/1 : spsSeriesRLCBranchLib/Series RLC Branch  LConnTagsString=__new0  RConnTagsString=__new0  BranchType=R  Resistance=(Rg_matrix(4,4)+Rg_matrix(3,4))*2  Inductance=1e-3  SetiL0=off  InitialCurrent=0  Capacitance=Rg_matrix(1,2)*2  Setx0=off  InitialVoltage=0  Measurements=None
  Rgsg1/2 : spsSeriesRLCBranchLib/Series RLC Branch  LConnTagsString=__new0  RConnTagsString=__new0  BranchType=R  Resistance=(Rg_matrix(2,2)+Rg_matrix(1,2))*2  Inductance=1e-3  SetiL0=off  InitialCurrent=0  Capacitance=Rg_matrix(1,2)*2  Setx0=off  InitialVoltage=0  Measurements=None
  Rgsg1/3 : spsSeriesRLCBranchLib/Series RLC Branch  LConnTagsString=__new0  RConnTagsString=__new0  BranchType=R  Resistance=(Rg_matrix(4,4)+Rg_matrix(3,4))*2  Inductance=1e-3  SetiL0=off  InitialCurrent=0  Capacitance=Rg_matrix(1,2)*2  Setx0=off  InitialVoltage=0  Measurements=None
  Rgsg1/4 : spsSeriesRLCBranchLib/Series RLC Branch  LConnTagsString=__new0  RConnTagsString=__new0  BranchType=R  Resistance=(Rg_matrix(2,2)+Rg_matrix(1,2))*2  Inductance=1e-3  SetiL0=off  InitialCurrent=0  Capacitance=Rg_matrix(1,2)*2  Setx0=off  InitialVoltage=0  Measurements=None
  Rsg*2 : spsSeriesRLCBranchLib/Series RLC Branch  LConnTagsString=__new0  RConnTagsString=__new0  BranchType=R  Resistance=(Rg_matrix(6,6)+Rg_matrix(5,6))*2  Inductance=1e-3  SetiL0=off  InitialCurrent=0  Capacitance=Rg_matrix(1,2)*2  Setx0=off  InitialVoltage=0  Measurements=None
  Rsg1/1 : spsSeriesRLCBranchLib/Series RLC Branch  LConnTagsString=__new0  RConnTagsString=__new0  BranchType=R  Resistance=(Rg_matrix(6,6)+Rg_matrix(5,6))*2  Inductance=1e-3  SetiL0=off  InitialCurrent=0  Capacitance=Rg_matrix(1,2)*2  Setx0=off  InitialVoltage=0  Measurements=None
  A : PMIOPort  Side=Left
  B : PMIOPort  Port=2  Side=Left
  C : PMIOPort  Port=3  Side=Left
  a : PMIOPort  Port=4  Side=Right
  b : PMIOPort  Port=5  Side=Right
  c : PMIOPort  Port=6  Side=Right
  connections:
  RL/LConn6 -- Ground3/LConn1 -- Rgsg1/2/LConn1 -- Csg/2/LConn1 -- Rcs*2/LConn1 -- Ccs/2/LConn1 -- RL/LConn2 -- RL/LConn4 -- Rgsg1/1/LConn1 -- Csg2/2/LConn1 -- Ccs2/3/LConn1 -- Ccs2/2/LConn1 -- Rsg*2/LConn1 -- Csg3/2/LConn1 -- Ccs3/3/LConn1 -- Ccs3/2/LConn1
  Rsg1/1/RConn1 -- Rgsg1/3/RConn1 -- Rgsg1/4/RConn1 -- Csg3/1/RConn1 -- Csg2/1/RConn1 -- Ground2/LConn1 -- Csg1/1/RConn1
  Rgsg1/3/LConn1 -- Ccs2/4/LConn1 -- Csg2/1/LConn1 -- Ccs2/1/LConn1 -- RL/RConn4 -- Rgsg1/4/LConn1 -- Rgcs1/1/LConn1 -- Csg1/1/LConn1 -- Ccs/1/LConn1 -- RL/RConn2 -- Ground4/LConn1 -- RL/RConn6 -- Ccs3/1/LConn1 -- Rsg1/1/LConn1 -- Ccs3/4/LConn1 -- Csg3/1/LConn1
  Rsg*2/RConn1 -- Rgsg1/1/RConn1 -- Rgsg1/2/RConn1 -- Csg3/2/RConn1 -- Csg2/2/RConn1 -- Ground1/LConn1 -- Csg/2/RConn1
  a/RConn1 -- RL/RConn1 -- Rgcs1/1/RConn1 -- Ccs/1/RConn1
  b/RConn1 -- RL/RConn3 -- Ccs2/4/RConn1 -- Ccs2/1/RConn1
  Ccs3/1/RConn1 -- c/RConn1 -- RL/RConn5 -- Ccs3/4/RConn1
  RL/LConn1 -- A/RConn1 -- Rcs*2/RConn1 -- Ccs/2/RConn1
  RL/LConn3 -- B/RConn1 -- Ccs2/3/RConn1 -- Ccs2/2/RConn1
  Ccs3/2/RConn1 -- C/RConn1 -- RL/LConn5 -- Ccs3/3/RConn1

== system SPGF_FSK_0000_R2022b/W34/DPL ==
  Ccs2/1 : spsSeriesRLCBranchLib/Series RLC Branch  LConnTagsString=__new0  RConnTagsString=__new0  BranchType=R  Resistance=-Rg_matrix(3,4)*2  Inductance=1e-3  SetiL0=off  InitialCurrent=0  Capacitance=Rg_matrix(3,4)*2  Setx0=off  InitialVoltage=0  Measurements=None
  Ccs2/3 : spsSeriesRLCBranchLib/Series RLC Branch  LConnTagsString=__new0  RConnTagsString=__new0  BranchType=R  Resistance=-Rg_matrix(3,4)*2  Inductance=1e-3  SetiL0=off  InitialCurrent=0  Capacitance=Rg_matrix(3,4)*2  Setx0=off  InitialVoltage=0  Measurements=None
  Ccs3/1 : spsSeriesRLCBranchLib/Series RLC Branch  LConnTagsString=__new0  RConnTagsString=__new0  BranchType=R  Resistance=-Rg_matrix(5,6)*2  Inductance=1e-3  SetiL0=off  InitialCurrent=0  Capacitance=-C_matrix(5,6)/2  Setx0=off  InitialVoltage=0  Measurements=None
  Ccs3/3 : spsSeriesRLCBranchLib/Series RLC Branch  LConnTagsString=__new0  RConnTagsString=__new0  BranchType=R  Resistance=-Rg_matrix(5,6)*2  Inductance=1e-3  SetiL0=off  InitialCurrent=0  Capacitance=-C_matrix(5,6)/2  Setx0=off  InitialVoltage=0  Measurements=None
  DPL : spsDistributedParametersLineLib/Distributed Parameters Line  Phases=6  Length=LineLength  Frequency=Frequency  Resistance=R_matrix  Inductance=L_matrix  Capacitance=C_matrix  x1=[-1.4e-05 -0.972688180508992 0 0 0 0 0;-1.35e-05 -0.9729628695725 0 0 0 0 0;-1.3e-05 -0.973237534629112 0 0 0 0 0;-1.25e-05 -0.973512175672049 0 0 0 0 0;-1.2e-05 -0.973786792694537 0 0 0 0 0;-1.15e-05 -0.974061385689799 0 0 0 0 0;-1.1e-05 -0.974335954651059 0 0 0 0 0;-1.05e-05 -0.974610499571544 0 0 0 0 0;-1e-05 -0.974885020444478 0 0 0 0 0;-9.5e-06 -0.975159517263089 0 0 0 0 0;-9e-06 -0.975433990020603 0 0 0 0 0;-8.5e-06 -0.975708438710248 0 0 0 0 0;-8e-06 -0.975982863325252 0 0 0 0 0;-7.5e-06 -0.976257263858845 0 0 0 0 0;-7e-06 -0.976531640304255 0 0 0 0 0;-6.5e-06 -0.976805992654713 0 0 0 0 0;-6e-06 -0.977080320903449 0 0 0 0 0;-5.5e-06 -0.977354625043694 0 0 0 0 0;-5e-06 -0.977628905068681 0 0 0 0 0;-4.5e-06 -0.977903160971641 0 0 0 0 0;-4e-06 -0.978177392745808 0 0 0 0 0;-3.5e-06 -0.978451600384416 0 -12.1380036408067 0 0 0;-3e-06 -0.978725783880698 0 -12.1414267667825 0 0 0;-2.5e-06 -0.978999943227889 4689.27287205568 -12.1448495931806 -2646.58058547797 0 -4667.80620468307;-2e-06 -0.979274078419225 4690.57135464546 -12.1482721199166 -2647.31343658441 -8267.30614902919 -4667.38938878142;-1.5e-06 -0.979548189447941 4691.86972150002 -12.151694346906 -2648.04622237101 -8266.56764266746 -4666.97245771656;-1e-06 -0.979822276307275 4693.16797258734 -12.1551162740643 -2648.77894281968 -8265.82893233636 -4666.55541149877;-5e-07 -0.980096338990463 4694.46610787538 -12.1585379013072 -2649.51159791236 -8265.09001805409 -4666.13825013833]  x2=[-1.4e-05 -0.972363344326687 0 0 0 0 0;-1.35e-05 -0.972639185382002 0 0 0 0 0;-1.3e-05 -0.972915002438407 0 0 0 0 0;-1.25e-05 -0.973190795489096 0 0 0 0 0;-1.2e-05 -0.973466564527265 0 0 0 0 0;-1.15e-05 -0.973742309546109 0 0 0 0 0;-1.1e-05 -0.974018030538825 0 0 0 0 0;-1.05e-05 -0.97429372749861 0 0 0 0 0;-1e-05 -0.97456940041866 0 0 0 0 0;-9.5e-06 -0.974845049292174 0 0 0 0 0;-9e-06 -0.975120674112351 0 0 0 0 0;-8.5e-06 -0.975396274872389 0 0 0 0 0;-8e-06 -0.97567185156549 0 0 0 0 0;-7.5e-06 -0.975947404184852 0 0 0 0 0;-7e-06 -0.976222932723677 0 0 0 0 0;-6.5e-06 -0.976498437175167 0 0 0 0 0;-6e-06 -0.976773917532524 0 0 0 0 0;-5.5e-06 -0.977049373788951 0 0 0 0 0;-5e-06 -0.97732480593765 0 0 0 0 0;-4.5e-06 -0.977600213971827 0 0 0 0 0;-4e-06 -0.977875597884685 0 0 0 0 0;-3.5e-06 -0.97815095766943 0 -12.1301398779662 0 0 0;-3e-06 -0.978426293319268 0 -12.1335812205604 0 0 0;-2.5e-06 -0.978701604827404 4690.60736458868 -12.1370222637705 -2647.33376025011 0 -4678.05550222133;-2e-06 -0.978976892187047 4691.90873795942 -12.1404630075116 -2648.06824288557 -8285.46059401154 -4677.63866010904;-1.5e-06 -0.979252155391403 4693.20999556194 -12.1439034516988 -2648.80266018256 -8284.72204077517 -4677.22170258063;-1e-06 -0.97952739443368 4694.51113736415 -12.1473435962471 -2649.53701212297 -8283.98328312148 -4676.80462964641;-5e-07 -0.979802609307088 4695.81216333394 -12.1507834410718 -2650.27129868867 -8283.2443210687 -4676.38744131665]  x3=[-1.4e-05 0.00307008409438484 0 0 0 0 0;-1.35e-05 0.00306803437628129 0 0 0 0 0;-1.3e-05 0.00306598458247704 0 0 0 0 0;-1.25e-05 0.00306393471302264 0 0 0 0 0;-1.2e-05 0.00306188476796869 0 0 0 0 0;-1.15e-05 0.00305983474736575 0 0 0 0 0;-1.1e-05 0.00305778465126443 0 0 0 0 0;-1.05e-05 0.00305573447971529 0 0 0 0 0;-1e-05 0.00305368423276892 0 0 0 0 0;-9.5e-06 0.00305163391047591 0 0 0 0 0;-9e-06 0.00304958351288686 0 0 0 0 0;-8.5e-06 0.00304753304005235 0 0 0 0 0;-8e-06 0.00304548249202298 0 0 0 0 0;-7.5e-06 0.00304343186884934 0 0 0 0 0;-7e-06 0.00304138117058202 0 0 0 0 0;-6.5e-06 0.00303933039727164 0 0 0 0 0;-6e-06 0.00303727954896878 0 0 0 0 0;-5.5e-06 0.00303522862572406 0 0 0 0 0;-5e-06 0.00303317762758806 0 0 0 0 0;-4.5e-06 0.00303112655461142 0 0 0 0 0;-4e-06 0.00302907540684472 0 0 0 0 0;-3.5e-06 0.00302702418433858 0 -0.517922252215807 0 0 0;-3e-06 0.00302497288714362 0 -0.518166847545212 0 0 0;-2.5e-06 0.00302292151531044 35.166775732862 -0.518411430089364 -188.360680344721 0 -395.80487756782;-2e-06 0.00302087006888966 35.1926548416718 -0.518655999842225 -188.41915581126 -180.794915832926 -395.773400192006;-1.5e-06 0.0030188185479319 35.2185330821378 -0.518900556797763 -188.477626628742 -180.787776725212 -395.741913050875;-1e-06 0.00301676695248778 35.2444104536213 -0.519145100949943 -188.536092795726 -180.780633156738 -395.710416145204;-5e-07 0.00301471528260791 35.2702869554838 -0.519389632292731 -188.594554310767 -180.77348512768 -395.678909475769]  x4=[-1.4e-05 -0.0143556629284314 0 0 0 0 0;-1.35e-05 -0.0143568240065626 0 0 0 0 0;-1.3e-05 -0.0143579847304534 0 0 0 0 0;-1.25e-05 -0.014359145100075 0 0 0 0 0;-1.2e-05 -0.014360305115399 0 0 0 0 0;-1.15e-05 -0.0143614647763967 0 0 0 0 0;-1.1e-05 -0.0143626240830394 0 0 0 0 0;-1.05e-05 -0.0143637830352986 0 0 0 0 0;-1e-05 -0.0143649416331456 0 0 0 0 0;-9.5e-06 -0.014366099876552 0 0 0 0 0;-9e-06 -0.014367257765489 0 0 0 0 0;-8.5e-06 -0.0143684152999281 0 0 0 0 0;-8e-06 -0.0143695724798408 0 0 0 0 0;-7.5e-06 -0.0143707293051985 0 0 0 0 0;-7e-06 -0.0143718857759727 0 0 0 0 0;-6.5e-06 -0.0143730418921348 0 0 0 0 0;-6e-06 -0.0143741976536563 0 0 0 0 0;-5.5e-06 -0.0143753530605087 0 0 0 0 0;-5e-06 -0.0143765081126635 0 0 0 0 0;-4.5e-06 -0.0143776628100921 0 0 0 0 0;-4e-06 -0.0143788171527662 0 0 0 0 0;-3.5e-06 -0.0143799711406572 0 -0.666584704633844 0 0 0;-3e-06 -0.0143811247737366 0 -0.666675531603208 0 0 0;-2.5e-06 -0.0143822780519759 66.7362978556831 -0.666766342123012 -185.775819327895 0 -313.387409901167;-2e-06 -0.0143834309753468 66.7386875041615 -0.666857136191017 -185.821132159976 -30.3342917504747 -313.355676409403;-1.5e-06 -0.0143845835438208 66.7410755059289 -0.666947913804981 -185.866440407105 -30.3226046530858 -313.323935185897;-1e-06 -0.0143857357573693 66.7434618609262 -0.667038674962665 -185.911744068163 -30.3109168075165 -313.292186231433;-5e-07 -0.0143868876159641 66.7458465690946 -0.667129419661829 -185.957043142032 -30.2992282140554 -313.260429546794]  x5=1.38995450716387e-05  V1=ones(3,3)  V2=ones(3,3)  I1=ones(3,3)  I2=ones(3,3)  nHarmo=1  Measurements=None  Decoupling=off  VsMag0=0  VrMag0=0  VsAngle0=0  VrAngle0=0  IsMag0=0  IrMag0=0  IsAngle0=0  IrAngle0=0
      settings: LibrarySourceBlock=sps_lib/Power Grid Elements/Distributed Parameters Line
  Ground{1..4} (4 alike) : spsGroundLib/Ground  LConnTagsString=a
  Rcs*1 : spsSeriesRLCBranchLib/Series RLC Branch  LConnTagsString=__new0  RConnTagsString=__new0  BranchType=R  Resistance=-Rg_matrix(1,2)*2  Inductance=1e-3  SetiL0=off  InitialCurrent=0  Capacitance=Rg_matrix(1,2)*2  Setx0=off  InitialVoltage=0  Measurements=None
  Rcs*2 : spsSeriesRLCBranchLib/Series RLC Branch  LConnTagsString=__new0  RConnTagsString=__new0  BranchType=R  Resistance=-Rg_matrix(1,2)*2  Inductance=1e-3  SetiL0=off  InitialCurrent=0  Capacitance=Rg_matrix(1,2)*2  Setx0=off  InitialVoltage=0  Measurements=None
  Rgsg1/1 : spsSeriesRLCBranchLib/Series RLC Branch  LConnTagsString=__new0  RConnTagsString=__new0  BranchType=R  Resistance=(Rg_matrix(4,4)+Rg_matrix(3,4))*2  Inductance=1e-3  SetiL0=off  InitialCurrent=0  Capacitance=Rg_matrix(1,2)*2  Setx0=off  InitialVoltage=0  Measurements=None
  Rgsg1/2 : spsSeriesRLCBranchLib/Series RLC Branch  LConnTagsString=__new0  RConnTagsString=__new0  BranchType=R  Resistance=(Rg_matrix(2,2)+Rg_matrix(1,2))*2  Inductance=1e-3  SetiL0=off  InitialCurrent=0  Capacitance=Rg_matrix(1,2)*2  Setx0=off  InitialVoltage=0  Measurements=None
  Rgsg1/3 : spsSeriesRLCBranchLib/Series RLC Branch  LConnTagsString=__new0  RConnTagsString=__new0  BranchType=R  Resistance=(Rg_matrix(4,4)+Rg_matrix(3,4))*2  Inductance=1e-3  SetiL0=off  InitialCurrent=0  Capacitance=Rg_matrix(1,2)*2  Setx0=off  InitialVoltage=0  Measurements=None
  Rgsg1/4 : spsSeriesRLCBranchLib/Series RLC Branch  LConnTagsString=__new0  RConnTagsString=__new0  BranchType=R  Resistance=(Rg_matrix(2,2)+Rg_matrix(1,2))*2  Inductance=1e-3  SetiL0=off  InitialCurrent=0  Capacitance=Rg_matrix(1,2)*2  Setx0=off  InitialVoltage=0  Measurements=None
  Rsg*1 : spsSeriesRLCBranchLib/Series RLC Branch  LConnTagsString=__new0  RConnTagsString=__new0  BranchType=R  Resistance=(Rg_matrix(6,6)+Rg_matrix(5,6))*2  Inductance=1e-3  SetiL0=off  InitialCurrent=0  Capacitance=Rg_matrix(1,2)*2  Setx0=off  InitialVoltage=0  Measurements=None
  Rsg*2 : spsSeriesRLCBranchLib/Series RLC Branch  LConnTagsString=__new0  RConnTagsString=__new0  BranchType=R  Resistance=(Rg_matrix(6,6)+Rg_matrix(5,6))*2  Inductance=1e-3  SetiL0=off  InitialCurrent=0  Capacitance=Rg_matrix(1,2)*2  Setx0=off  InitialVoltage=0  Measurements=None
  A : PMIOPort  Side=Left
  B : PMIOPort  Port=2  Side=Left
  C : PMIOPort  Port=3  Side=Left
  a : PMIOPort  Port=4  Side=Right
  b : PMIOPort  Port=5  Side=Right
  c : PMIOPort  Port=6  Side=Right
  connections:
  c/RConn1 -- Ccs3/1/RConn1 -- DPL/RConn5
  b/RConn1 -- Ccs2/1/RConn1 -- DPL/RConn3
  a/RConn1 -- DPL/RConn1 -- Rcs*1/RConn1
  Ground4/LConn1 -- DPL/RConn6 -- Ccs3/1/LConn1 -- Rsg*1/LConn1 -- Rcs*1/LConn1 -- Rgsg1/4/LConn1 -- DPL/RConn2 -- DPL/RConn4 -- Ccs2/1/LConn1 -- Rgsg1/3/LConn1
  Ground1/LConn1 -- Rgsg1/4/RConn1 -- Rsg*1/RConn1 -- Rgsg1/3/RConn1
  Ground3/LConn1 -- Ccs3/3/LConn1 -- Rsg*2/LConn1 -- DPL/LConn6 -- Rgsg1/1/LConn1 -- Ccs2/3/LConn1 -- DPL/LConn4 -- Rgsg1/2/LConn1 -- Rcs*2/LConn1 -- DPL/LConn2
  Ground2/LConn1 -- Rgsg1/1/RConn1 -- Rsg*2/RConn1 -- Rgsg1/2/RConn1
  Ccs3/3/RConn1 -- DPL/LConn5 -- C/RConn1
  Ccs2/3/RConn1 -- DPL/LConn3 -- B/RConn1
  Rcs*2/RConn1 -- DPL/LConn1 -- A/RConn1
